simulink model "controlador_smc_diag"  (R2018b)
settings: Solver=ode23s  StartTime=0.0  StopTime=10.0  MaxStep=0.05  MinStep=0.0001  RelTol=1e-3
values from neighbouring files (symbols this model uses):
  k1 = lambda^2    [sliding_mode.m]
  k2 = 2*lambda    [sliding_mode.m]
  lambda = 10    [sliding_mode.m]
  ref = 0.09    [sliding_mode.m]
  x0 = [0.005; 0; 0.5]    [sliding_mode.m]
settings Model: Creator=User  LastModifiedBy=User

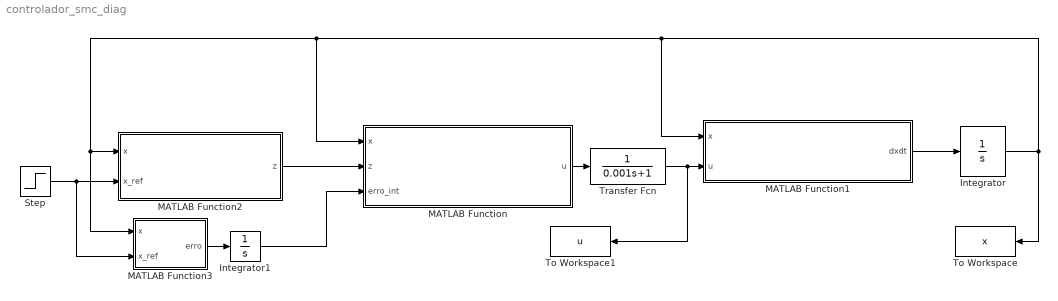
== system controlador_smc_diag ==
  Integrator : Integrator  InitialCondition=x0
  Integrator1 : Integrator
  MATLAB Function : MATLAB Function  TreatAsAtomicUnit=on
  MATLAB Function1 : MATLAB Function  TreatAsAtomicUnit=on
  MATLAB Function2 : MATLAB Function  TreatAsAtomicUnit=on
  MATLAB Function3 : MATLAB Function  TreatAsAtomicUnit=on
  Step : Step  Time=4  Before=0.015  After=ref  SampleTime=0
  To Workspace : ToWorkspace  VariableName=x  SaveFormat=Timeseries  SampleTime=-1
  To Workspace1 : ToWorkspace  VariableName=u  SaveFormat=Timeseries  SampleTime=-1
  Transfer Fcn : TransferFcn  Denominator=[0.001 1]
  wires:
  MATLAB Function1/1(dxdt) -> Integrator/1
  Integrator/1 -> To Workspace/1, MATLAB Function1/1(x), MATLAB Function3/1(x), MATLAB Function2/1(x), MATLAB Function/1(x)
  Step/1 -> MATLAB Function3/2(x_ref), MATLAB Function2/2(x_ref)
  MATLAB Function/1(u) -> Transfer Fcn/1
  Transfer Fcn/1 -> To Workspace1/1, MATLAB Function1/2(u)
  MATLAB Function2/1(z) -> MATLAB Function/2(z)
  MATLAB Function3/1(erro) -> Integrator1/1
  Integrator1/1 -> MATLAB Function/3(erro_int)

== matlab function controlador_smc_diag/MATLAB Function1 ==
  settings: updateMethod=CONTINUOUS  sampleTime=0
  data: x input; u input; dxdt output; paramsr parameter
function dxdt = planta_mls(x, u, paramsr)
    x1 = x(1); x2 = x(2); x3 = x(3);
    params = pn();

    b_nom  = [paramsr.b3, paramsr.b2, paramsr.b1, paramsr.b0];
    Px   = @(y) polyval(b_nom, y);
    
    % Equações de Estado
    dx1 = x2;
    dx2 = paramsr.g - (x3^2)/(paramsr.m * Px(x1));
    dx3 = (1/paramsr.L0) * (u - paramsr.R*x3 - x3*(2/Px(x1))*x2);
    
    dxdt = [dx1; dx2; dx3];
end

== matlab function controlador_smc_diag/MATLAB Function ==
  settings: updateMethod=CONTINUOUS
  data: x input; u output; z input; erro_int input; k1 parameter; k2 parameter; lambda parameter
function u = controlador_inv_dinamica(x, z, erro_int, k1, k2, lambda)
    % x = [posicao; velocidade; corrente]
    % v = sinal do controlador linear
    % params = struct com m, g, R, L0, b0, b1, b2, b3
    params = pn();
    x1 = x(1); x2 = x(2); x3 = x(3);
    b_nom  = [params.b3, params.b2, params.b1, params.b0];
    % Polinômio Denominador e sua derivada
    Px   = @(y) polyval(b_nom, y);
    dPx  = @(y) polyval(polyder(b_nom), y);
    
    % Cálculo de LgLf2h (Ganho de controle)
    LgLf2h = -(2 * x3) / (params.L0 * params.m * Px(x1));
    
    % Cálculo de Lf3h (Dinâmica livre)
    term1 = (2*x3 * (params.R*x3 + (2*x2*x3)/Px(x1))) / (params.L0 * params.m * Px(x1));
    term2 = (x2 * x3^2 * dPx(x1)) / (params.m * Px(x1)^2);
    Lf3h = term1 + term2;
    
    % Lei de Controle por Inversão com proteção contra singularidade
    % Se x3 estiver perto de zero, o ganho de controle some.
    % Usamos um limite inferior para LgLf2h
    if abs(LgLf2h) < 1e-4
        Lg_safe = -1e-4; % Mantém o sinal negativo
    else
        Lg_safe = LgLf2h;
    end
    
    beta = 200;
    mu = 0.05;
%     Para SMC
%     Termo Equivalente + Termo de Robustez
%     s = z(3) + k2*z(2) + k1*z(1);
%     u_eq = -(Lf3h + k2*z(3) + k1*z(2)) / Lg_safe;
    
%     Para ISMC
    % SUPERFÍCIE INTEGRAL (ISMC)
    s = z(3) + 3*lambda*z(2) + 3*lambda^2*z(1) + lambda^3*erro_int;
    % LEI DE CONTROLE
    % Note que agora u_eq precisa compensar o novo termo integral (lambda^3 * e)
    u_eq = -(Lf3h + 3*lambda*z(3) + 3*lambda^2*z(2) + lambda^3*z(1)) / Lg_safe;  
    
    u_n  = -(beta / Lg_safe) * max(min(s/mu, 1), -1); % sat(s/mu)
    
    u = u_eq + u_n;
    
    % Saturação física (Tabela I do artigo: 5V)
    if u > 5, u = 5; end
    if u < -5, u = -5; end
end

== matlab function controlador_smc_diag/MATLAB Function2 ==
  settings: updateMethod=CONTINUOUS
  data: x input; z output; x_ref input
function z = coord_transform(x, x_ref)
    % z1 = erro de posição
    % z2 = velocidade (derivada do erro)
    % z3 = aceleração não linear (segunda derivada do erro)
    params = pn();
    x1 = x(1); x2 = x(2); x3 = x(3);
    b_nom  = [params.b3, params.b2, params.b1, params.b0];
    % Polinômio Denominador e sua derivada
    Px   = @(y) polyval(b_nom, y);
    
    z1 = x1 - x_ref;
    z2 = x2;
    z3 = params.g - (x3^2)/(params.m * Px(x1)); % Lf^2 h
    
    z = [z1; z2; z3];
end

== matlab function controlador_smc_diag/MATLAB Function3 ==
  data: x input; erro output; x_ref input
function erro = fcn(x, x_ref)

erro = x(1) - x_ref;
